simulink model "CuantizadorS"  (R2016a)
settings: Solver=VariableStepAuto  StartTime=0.0  StopTime=10.0  RelTol=1e-3
settings Model: Creator=Anselmo  LastModifiedBy=Anselmo

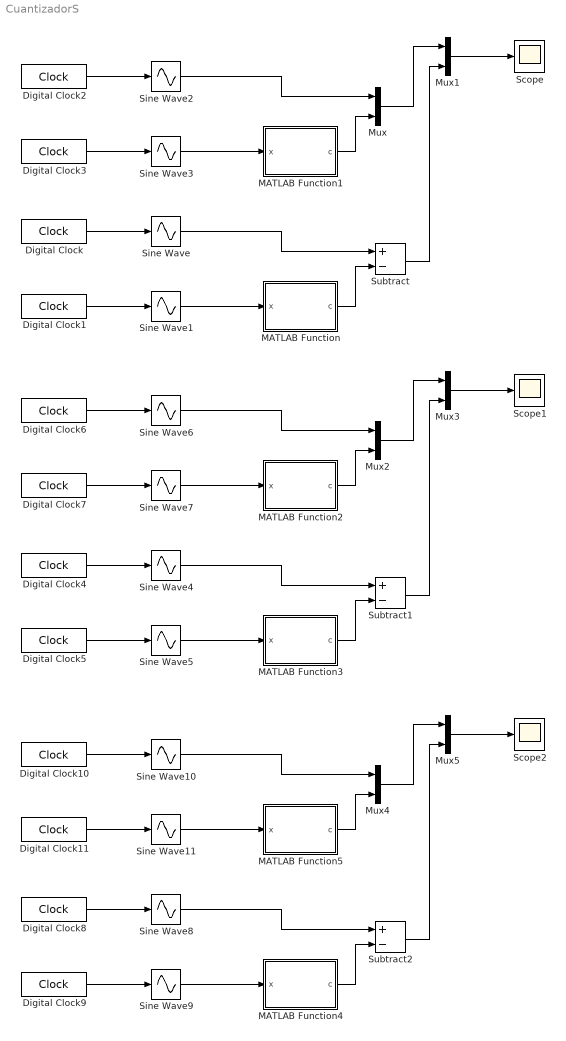
== system CuantizadorS ==
  Digital Clock{,1..11} (12 alike) : DigitalClock  SampleTime=0.001
  MATLAB Function : MATLAB Function  TreatAsAtomicUnit=on
  MATLAB Function1 : MATLAB Function  TreatAsAtomicUnit=on
  MATLAB Function2 : MATLAB Function  TreatAsAtomicUnit=on
  MATLAB Function3 : MATLAB Function  TreatAsAtomicUnit=on
  MATLAB Function4 : MATLAB Function  TreatAsAtomicUnit=on
  MATLAB Function5 : MATLAB Function  TreatAsAtomicUnit=on
  Mux{,1..5} (6 alike) : Mux  Inputs=2
  Scope : Scope
  Scope1 : Scope
  Scope2 : Scope
  Sine Wave{,1..11} (12 alike) : Sin  SineType=Sample based  TimeSource=Use external signal  Samples=4000  SampleTime=0
  Subtract : Sum  Inputs=+-
  Subtract1 : Sum  Inputs=+-
  Subtract2 : Sum  Inputs=+-
  wires:
  Digital Clock/1 -> Sine Wave/1
  Digital Clock1/1 -> Sine Wave1/1
  Sine Wave1/1 -> MATLAB Function/1(x)
  Sine Wave/1 -> Subtract/1
  MATLAB Function/1(c) -> Subtract/2
  Digital Clock2/1 -> Sine Wave2/1
  Digital Clock3/1 -> Sine Wave3/1
  Sine Wave3/1 -> MATLAB Function1/1(x)
  Sine Wave2/1 -> Mux/1
  MATLAB Function1/1(c) -> Mux/2
  Mux1/1 -> Scope/1
  Mux/1 -> Mux1/1
  Subtract/1 -> Mux1/2
  Digital Clock4/1 -> Sine Wave4/1
  Digital Clock5/1 -> Sine Wave5/1
  Sine Wave5/1 -> MATLAB Function3/1(x)
  Sine Wave4/1 -> Subtract1/1
  MATLAB Function3/1(c) -> Subtract1/2
  Digital Clock6/1 -> Sine Wave6/1
  Digital Clock7/1 -> Sine Wave7/1
  Sine Wave7/1 -> MATLAB Function2/1(x)
  Sine Wave6/1 -> Mux2/1
  MATLAB Function2/1(c) -> Mux2/2
  Mux3/1 -> Scope1/1
  Mux2/1 -> Mux3/1
  Subtract1/1 -> Mux3/2
  Digital Clock8/1 -> Sine Wave8/1
  Digital Clock9/1 -> Sine Wave9/1
  Sine Wave9/1 -> MATLAB Function4/1(x)
  Sine Wave8/1 -> Subtract2/1
  MATLAB Function4/1(c) -> Subtract2/2
  Digital Clock10/1 -> Sine Wave10/1
  Digital Clock11/1 -> Sine Wave11/1
  Sine Wave11/1 -> MATLAB Function5/1(x)
  Sine Wave10/1 -> Mux4/1
  MATLAB Function5/1(c) -> Mux4/2
  Mux5/1 -> Scope2/1
  Mux4/1 -> Mux5/1
  Subtract2/1 -> Mux5/2

== matlab function CuantizadorS/MATLAB Function1 ==
  data: x input; c output
function c=Cuantizador(x)
    L=8;
    x_max=1;
    escalon=(2*x_max)/L;
    y=zeros(1,L+1);
    y(1)=-x_max;
    Y=zeros(1,L);
    
    for i=1:L
        y(i+1)=y(i)+escalon;
        Y(i)=(y(i)+y(i+1))/2;
    end
    
    sig=0;
    for i=1:length(y)
        if(x>=y(length(y)))
            sig=Y(length(Y));
        elseif(x<=y(1))
            sig=Y(1);
        elseif(x>=y(i)&&x<y(i+1))
            sig=Y(i);
        end
    end
    c=sig;

== matlab function CuantizadorS/MATLAB Function ==
  data: x input; c output
function c=Cuantizador(x)
    L=8;
    x_max=1;
    escalon=(2*x_max)/L;
    y=zeros(1,L+1);
    y(1)=-x_max;
    Y=zeros(1,L);
    
    for i=1:L
        y(i+1)=y(i)+escalon;
        Y(i)=(y(i)+y(i+1))/2;
    end
    
    sig=0;
    for i=1:length(y)
        if(x>=y(length(y)))
            sig=Y(length(Y));
        elseif(x<=y(1))
            sig=Y(1);
        elseif(x>=y(i)&&x<y(i+1))
            sig=Y(i);
        end
    end
    c=sig;

== matlab function CuantizadorS/MATLAB Function2 ==
  data: x input; c output
function c=Cuantizador(x)
    L=16;
    x_max=1;
    escalon=(2*x_max)/L;
    y=zeros(1,L+1);
    y(1)=-x_max;
    Y=zeros(1,L);
    
    for i=1:L
        y(i+1)=y(i)+escalon;
        Y(i)=(y(i)+y(i+1))/2;
    end
    
    sig=0;
    for i=1:length(y)
        if(x>=y(length(y)))
            sig=Y(length(Y));
        elseif(x<=y(1))
            sig=Y(1);
        elseif(x>=y(i)&&x<y(i+1))
            sig=Y(i);
        end
    end
    c=sig;

== matlab function CuantizadorS/MATLAB Function3 ==
  data: x input; c output
function c=Cuantizador(x)
    L=16;
    x_max=1;
    escalon=(2*x_max)/L;
    y=zeros(1,L+1);
    y(1)=-x_max;
    Y=zeros(1,L);
    
    for i=1:L
        y(i+1)=y(i)+escalon;
        Y(i)=(y(i)+y(i+1))/2;
    end
    
    sig=0;
    for i=1:length(y)
        if(x>=y(length(y)))
            sig=Y(length(Y));
        elseif(x<=y(1))
            sig=Y(1);
        elseif(x>=y(i)&&x<y(i+1))
            sig=Y(i);
        end
    end
    c=sig;

== matlab function CuantizadorS/MATLAB Function4 ==
  data: x input; c output
function c=Cuantizador(x)
    L=32;
    x_max=1;
    escalon=(2*x_max)/L;
    y=zeros(1,L+1);
    y(1)=-x_max;
    Y=zeros(1,L);
    
    for i=1:L
        y(i+1)=y(i)+escalon;
        Y(i)=(y(i)+y(i+1))/2;
    end
    
    sig=0;
    for i=1:length(y)
        if(x>=y(length(y)))
            sig=Y(length(Y));
        elseif(x<=y(1))
            sig=Y(1);
        elseif(x>=y(i)&&x<y(i+1))
            sig=Y(i);
        end
    end
    c=sig;

== matlab function CuantizadorS/MATLAB Function5 ==
  data: x input; c output
function c=Cuantizador(x)
    L=32;
    x_max=1;
    escalon=(2*x_max)/L;
    y=zeros(1,L+1);
    y(1)=-x_max;
    Y=zeros(1,L);
    
    for i=1:L
        y(i+1)=y(i)+escalon;
        Y(i)=(y(i)+y(i+1))/2;
    end
    
    sig=0;
    for i=1:length(y)
        if(x>=y(length(y)))
            sig=Y(length(Y));
        elseif(x<=y(1))
            sig=Y(1);
        elseif(x>=y(i)&&x<y(i+1))
            sig=Y(i);
        end
    end
    c=sig;
